simulink model "PI"  (R2016b)
settings: Solver=VariableStepAuto  StartTime=0.0  StopTime=10.0  RelTol=1e-3
undefined symbols (not defined in the file or in its folder): G
settings Model: Creator=Akash  LastModifiedBy=Akash

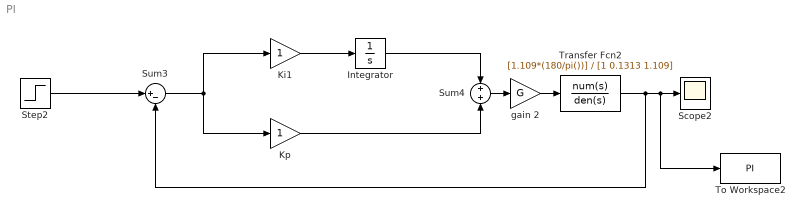
== system PI ==
  Integrator : Integrator
  Ki1 : Gain
  "Kp " : Gain
  Scope2 : Scope
  Step2 : Step  SampleTime=0
  Sum3 : Sum  Inputs=|+-
  Sum4 : Sum
  To Workspace2 : ToWorkspace  VariableName=PI  SaveFormat=Timeseries  SampleTime=-1
  Transfer Fcn2 : TransferFcn  Numerator=[1.109*(180/pi())]  Denominator=[1 0.1313 1.109]
  gain 2 : Gain  Gain=G
  wires:
  Step2/1 -> Sum3/1
  Sum3/1 -> "Kp "/1, Ki1/1
  Transfer Fcn2/1 -> Sum3/2, To Workspace2/1, Scope2/1
  Sum4/1 -> gain 2/1
  gain 2/1 -> Transfer Fcn2/1
  Ki1/1 -> Integrator/1
  "Kp "/1 -> Sum4/2
  Integrator/1 -> Sum4/1
